simulink model "Practica6"  (R2021a)
settings: Solver=FixedStepDiscrete  StartTime=0.0  StopTime=15.0  FixedStep=1  RelTol=1e-3
libraries: dspsrcs4 x4
settings Model: Creator=Diego  LastModifiedBy=Diego

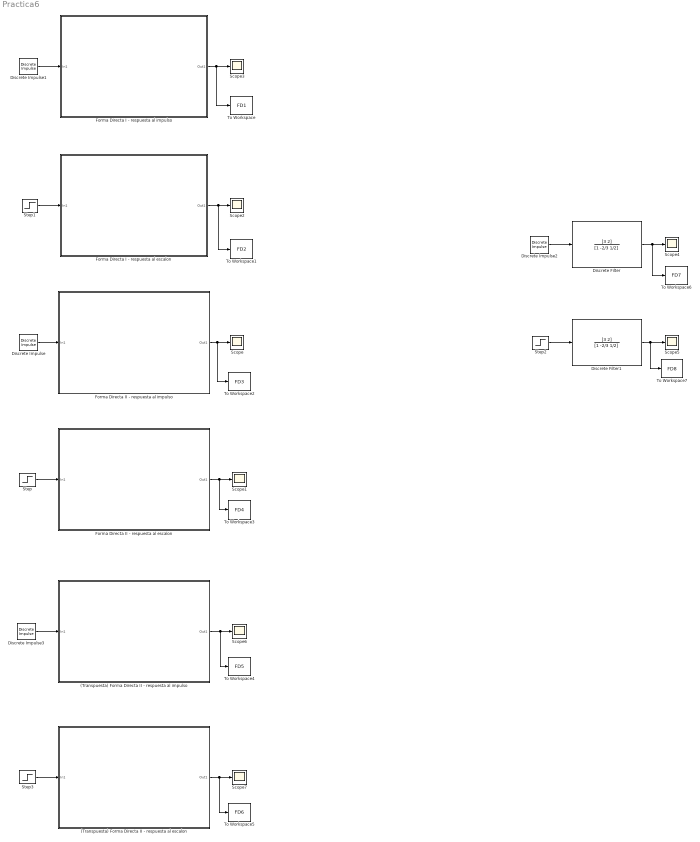
== system Practica6 ==
  (Transpuesta) Forma Directa II - respuesta al escalon : Subsystem
      mask Display: image('D:\5to Semestre\Procesamiento Digital\Practica 6\Capturas\Mascara-Transpuesta-FormaDirecta-II.jpeg'); % Use "Edit Image" on toolstrip to change.
  (Transpuesta) Forma Directa II - respuesta al impulso : Subsystem
      mask Display: image('D:\5to Semestre\Procesamiento Digital\Practica 6\Capturas\Mascara-Transpuesta-FormaDirecta-II.jpeg'); % Use "Edit Image" on toolstrip to change.
  Discrete Impulse{,1..3} (4 alike) : dspsrcs4/Discrete  Impulse  Delay=0  SampleTime=1  FrameSample=1  OutputFrames=off  dataType=double  isSigned=on  wordLen=16  udDataType=sfix(16)  fracBitsMode=Best precision  numFracBits=15  OutDataTypeStr=double  LastOutDataTypeStr=double
  Discrete Filter : DiscreteFilter  Numerator=[3 2]  Denominator=[1 -2/3 1/2]  FilterStructure=Direct form II transposed
  Discrete Filter1 : DiscreteFilter  Numerator=[3 2]  Denominator=[1 -2/3 1/2]  FilterStructure=Direct form II transposed
  Forma Directa I - respuesta al escalon : Subsystem
      mask Display: image('D:\5to Semestre\Procesamiento Digital\Practica 6\Capturas\Mascara-FormaDirecta-I.jpeg'); % Use "Edit Image" on toolstrip to change.
  Forma Directa I - respuesta al impulso : Subsystem
      mask Display: image('D:\5to Semestre\Procesamiento Digital\Practica 6\Capturas\Mascara-FormaDirecta-I.jpeg'); % Use "Edit Image" on toolstrip to change.
  Forma Directa II - respuesta al escalon : Subsystem
      mask Display: image('D:\5to Semestre\Procesamiento Digital\Practica 6\Capturas\Mascara-FormaDirecta-II.jpeg'); % Use "Edit Image" on toolstrip to change.
  Forma Directa II - respuesta al impulso : Subsystem
      mask Display: image('D:\5to Semestre\Procesamiento Digital\Practica 6\Capturas\Mascara-FormaDirecta-II.jpeg'); % Use "Edit Image" on toolstrip to change.
  Scope{,1..7} (8 alike) : Scope
  Step : Step  Time=0  SampleTime=1
  Step1 : Step  Time=0  SampleTime=1
  Step2 : Step  Time=0  SampleTime=1
  Step3 : Step  Time=0  SampleTime=0
  To Workspace : ToWorkspace  VariableName=FD1  SampleTime=-1
      settings: Save2DSignal=2-D array (concatenate along first dimension)
  To Workspace1 : ToWorkspace  VariableName=FD2  SampleTime=-1
      settings: Save2DSignal=2-D array (concatenate along first dimension)
  To Workspace2 : ToWorkspace  VariableName=FD3  SampleTime=-1
      settings: Save2DSignal=2-D array (concatenate along first dimension)
  To Workspace3 : ToWorkspace  VariableName=FD4  SampleTime=-1
      settings: Save2DSignal=2-D array (concatenate along first dimension)
  To Workspace4 : ToWorkspace  VariableName=FD5  SampleTime=-1
      settings: Save2DSignal=2-D array (concatenate along first dimension)
  To Workspace5 : ToWorkspace  VariableName=FD6  SampleTime=-1
      settings: Save2DSignal=2-D array (concatenate along first dimension)
  To Workspace6 : ToWorkspace  VariableName=FD7  SampleTime=-1
      settings: Save2DSignal=2-D array (concatenate along first dimension)
  To Workspace7 : ToWorkspace  VariableName=FD8  SampleTime=-1
      settings: Save2DSignal=2-D array (concatenate along first dimension)
  wires:
  Forma Directa II - respuesta al impulso/1(Out1) -> To Workspace2/1, Scope/1
  Discrete Impulse/1 -> Forma Directa II - respuesta al impulso/1(In1)
  Forma Directa II - respuesta al escalon/1(Out1) -> To Workspace3/1, Scope1/1
  Step/1 -> Forma Directa II - respuesta al escalon/1(In1)
  Step1/1 -> Forma Directa I - respuesta al escalon/1(In1)
  Forma Directa I - respuesta al escalon/1(Out1) -> To Workspace1/1, Scope2/1
  Discrete Impulse1/1 -> Forma Directa I - respuesta al impulso/1(In1)
  Discrete Impulse2/1 -> Discrete Filter/1
  Discrete Filter/1 -> To Workspace6/1, Scope4/1
  Step2/1 -> Discrete Filter1/1
  Discrete Impulse3/1 -> (Transpuesta) Forma Directa II - respuesta al impulso/1(In1)
  (Transpuesta) Forma Directa II - respuesta al impulso/1(Out1) -> To Workspace4/1, Scope6/1
  Step3/1 -> (Transpuesta) Forma Directa II - respuesta al escalon/1(In1)
  (Transpuesta) Forma Directa II - respuesta al escalon/1(Out1) -> To Workspace5/1, Scope7/1
  Forma Directa I - respuesta al impulso/1(Out1) -> Scope3/1, To Workspace/1
  Discrete Filter1/1 -> To Workspace7/1, Scope5/1

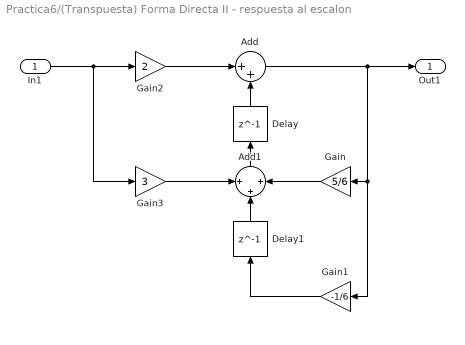
== system Practica6/(Transpuesta) Forma Directa II - respuesta al escalon ==
  In1 : Inport
  Add : Sum  Inputs=|++
  Add1 : Sum  Inputs=+|+|+
  Delay : Delay  DelayLength=1
  Delay1 : Delay  DelayLength=1
  Gain : Gain  Gain=5/6
  Gain1 : Gain  Gain=-1/6
  Gain2 : Gain  Gain=2
  Gain3 : Gain  Gain=3
  Out1 : Outport
  wires:
  Gain2/1 -> Add/1
  Gain3/1 -> Add1/1
  Add1/1 -> Delay/1
  In1/1 -> Gain3/1, Gain2/1
  Add/1 -> Out1/1, Gain1/1, Gain/1
  Gain/1 -> Add1/3
  Gain1/1 -> Delay1/1
  Delay/1 -> Add/2
  Delay1/1 -> Add1/2

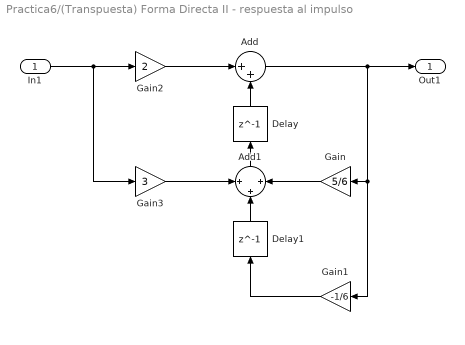
== system Practica6/(Transpuesta) Forma Directa II - respuesta al impulso ==
  In1 : Inport
  Add : Sum  Inputs=|++
  Add1 : Sum  Inputs=+|+|+
  Delay : Delay  DelayLength=1
  Delay1 : Delay  DelayLength=1
  Gain : Gain  Gain=5/6
  Gain1 : Gain  Gain=-1/6
  Gain2 : Gain  Gain=2
  Gain3 : Gain  Gain=3
  Out1 : Outport
  wires:
  Gain2/1 -> Add/1
  Gain3/1 -> Add1/1
  Add1/1 -> Delay/1
  In1/1 -> Gain3/1, Gain2/1
  Add/1 -> Out1/1, Gain1/1, Gain/1
  Gain/1 -> Add1/3
  Gain1/1 -> Delay1/1
  Delay/1 -> Add/2
  Delay1/1 -> Add1/2

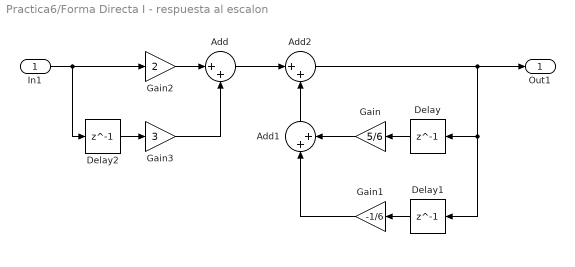
== system Practica6/Forma Directa I - respuesta al escalon ==
  In1 : Inport
  Add : Sum  Inputs=|++
  Add1 : Sum  Inputs=|++
  Add2 : Sum  Inputs=|++
  Delay : Delay  DelayLength=1
  Delay1 : Delay  DelayLength=1
  Delay2 : Delay  DelayLength=1
  Gain : Gain  Gain=5/6
  Gain1 : Gain  Gain=-1/6
  Gain2 : Gain  Gain=2
  Gain3 : Gain  Gain=3
  Out1 : Outport
  wires:
  Add1/1 -> Add2/2
  In1/1 -> Delay2/1, Gain2/1
  Add2/1 -> Out1/1, Delay1/1, Delay/1
  Gain1/1 -> Add1/1
  Delay2/1 -> Gain3/1
  Gain/1 -> Add1/2
  Delay1/1 -> Gain1/1
  Gain2/1 -> Add/1
  Gain3/1 -> Add/2
  Add/1 -> Add2/1
  Delay/1 -> Gain/1

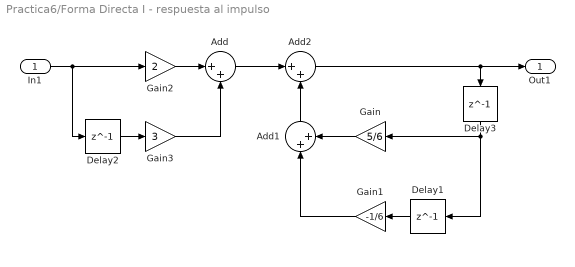
== system Practica6/Forma Directa I - respuesta al impulso ==
  In1 : Inport
  Add : Sum  Inputs=|++
  Add1 : Sum  Inputs=|++
  Add2 : Sum  Inputs=|++
  Delay1 : Delay  DelayLength=1
  Delay2 : Delay  DelayLength=1
  Delay3 : Delay  DelayLength=1
  Gain : Gain  Gain=5/6
  Gain1 : Gain  Gain=-1/6
  Gain2 : Gain  Gain=2
  Gain3 : Gain  Gain=3
  Out1 : Outport
  wires:
  Add1/1 -> Add2/2
  In1/1 -> Delay2/1, Gain2/1
  Add2/1 -> Delay3/1, Out1/1
  Gain1/1 -> Add1/1
  Delay2/1 -> Gain3/1
  Gain/1 -> Add1/2
  Delay1/1 -> Gain1/1
  Gain2/1 -> Add/1
  Gain3/1 -> Add/2
  Add/1 -> Add2/1
  Delay3/1 -> Delay1/1, Gain/1

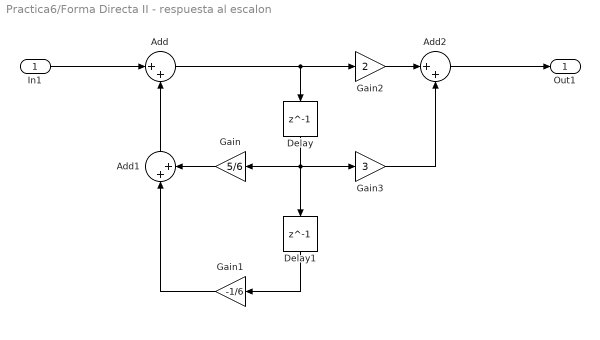
== system Practica6/Forma Directa II - respuesta al escalon ==
  In1 : Inport
  Add : Sum  Inputs=|++
  Add1 : Sum  Inputs=|++
  Add2 : Sum  Inputs=|++
  Delay : Delay  DelayLength=1
  Delay1 : Delay  DelayLength=1
  Gain : Gain  Gain=5/6
  Gain1 : Gain  Gain=-1/6
  Gain2 : Gain  Gain=2
  Gain3 : Gain  Gain=3
  Out1 : Outport
  wires:
  Delay1/1 -> Gain1/1
  Gain2/1 -> Add2/1
  Gain/1 -> Add1/2
  Delay/1 -> Gain/1, Gain3/1, Delay1/1
  In1/1 -> Add/1
  Add/1 -> Gain2/1, Delay/1
  Gain1/1 -> Add1/1
  Add2/1 -> Out1/1
  Gain3/1 -> Add2/2
  Add1/1 -> Add/2

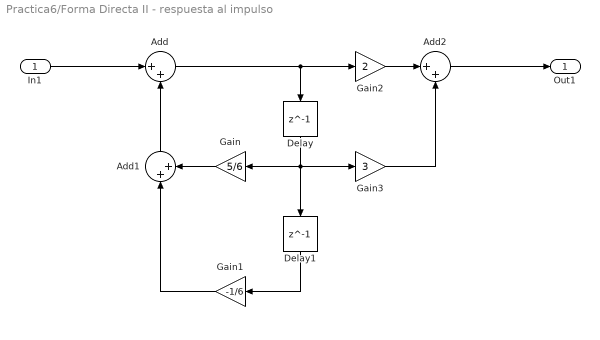
== system Practica6/Forma Directa II - respuesta al impulso ==
  In1 : Inport
  Add : Sum  Inputs=|++
  Add1 : Sum  Inputs=|++
  Add2 : Sum  Inputs=|++
  Delay : Delay  DelayLength=1
  Delay1 : Delay  DelayLength=1
  Gain : Gain  Gain=5/6
  Gain1 : Gain  Gain=-1/6
  Gain2 : Gain  Gain=2
  Gain3 : Gain  Gain=3
  Out1 : Outport
  wires:
  Delay1/1 -> Gain1/1
  Gain2/1 -> Add2/1
  Gain/1 -> Add1/2
  Delay/1 -> Gain/1, Gain3/1, Delay1/1
  In1/1 -> Add/1
  Add/1 -> Gain2/1, Delay/1
  Gain1/1 -> Add1/1
  Gain3/1 -> Add2/2
  Add2/1 -> Out1/1
  Add1/1 -> Add/2
